simulink library "GOcontroll_Moduline_Target"  (R2023b)
settings: Solver=ode45  StartTime=0.0  StopTime=10.0  RelTol=1e-3  EnableMultiTasking=on
PreLoadFcn:
  | compile_gocontroll_mex;
libraries: $bdroot x8, canmsglib x4, simulink x2
(part 2 of 4)

== system GOcontroll_Moduline_Target/Modules/Bridge Module ==
  Bridge Module : M-S-Function  FunctionName=sfcn_gocontroll_bridge_module  Parameters=tsamp  mask(Bridge Module){tsamp=1, ContrType=GOcontroll Moduline IV, moduleSlot=Moduleslot 1, C1func=Disable (output disabled), C1freq=100 Hz, C2func=Disable (output disabled), C2freq=100 Hz}
      mask prompts: tsamp "Sample time"; ContrType "Controller Type"; moduleSlot "Module Slot"; C1func "Function select"; C1freq "Frequency"; C2func "Function select"; C2freq "Frequency"
      mask help:
      | With this function block, you can configure each output of the bridge module (202001xx). During initialization of the controller, the corresponding outputs of the module are set according the settings. During runtime, the value pushed into the block will control the outputs.
      |
      | Module slot:
      | Sets the location of the module slot where the module is physically
      | plugged into.
      |
      | Channel tabs:
      | Each ouput has its own configuration tab.
      |
      | Function select:
      | Select the desired output configuration.
      |
      | Frequency:
      | In case a duty cycle is used, select the frequency.
      mask init:
      | % array with pinID infos
      | 	moduleSlotInfoStrings = {  	'Module Slot 1',  ...
      | 								'Module Slot 2',  ...
      | 								'Module Slot 3',  ...
      | 								'Module Slot 4',  ...
      | 								'Module Slot 5',  ...
      | 								'Module Slot 6',  ...
      | 								'Module Slot 7',  ...
      | 								'Module Slot 8'};
      | 	% construct the pinID info string
      | 	moduleSlotInfoStr = moduleSlotInfoStrings{moduleSlot};
      | 
      | 
      | 	if(moduleSlot == 1 || moduleSlot == 2)
      | 		connectorId = 'A';
      | 	elseif(moduleSlot == 3 || moduleSlot == 4)
      | 		connectorId = 'B';
      | 	elseif(moduleSlot == 5 || moduleSlot == 6)
      | 		connectorId = 'D';
      | 	else
      | 		connectorId = 'E';
      | 	end
      | 
      | 	if (ContrType == 1) % Moduline IV
      | 		if (mod(moduleSlot,2) == 1) %uneven
      | 			pin1Id = 'Pin 11,12,13';
      | 			pin2Id = 'Pin 17,18,19';
      | 		else
      | 			pin1Id = 'Pin 8,9,10';
      | 			pin2Id = 'Pin 14,15,16';
      | 		end
      | 	elseif(ContrType == 2 || ContrType == 3) % Moduline mini / Moduline display
      | 		if(mod(moduleSlot,2) == 1)
      | 			pin1Id = 'Pin 13,14,15';
      | 			pin2Id = 'Pin 21,22,23';
      | 		else
      | 			pin1Id = 'Pin 10,11,12';
      | 			pin2Id = 'Pin 18,19,20';
      | 		end
      |     end
      |     % register rtw data here because the WriteRTW callback doesn't update
      |     % properly
      |     % Create resource keywords to be reserved in resource database
      | 	modelRTWFields = 	struct('moduleSlot', int2str(moduleSlot),	'C1func', int2str(C1func),'C1freq', int2str(C1freq),...
      | 										'C2func', int2str(C2func),'C2freq', int2str(C2freq));
      | 
      | 	set_param(gcb, 'RTWdata', modelRTWFields);
      mask TypeOptions ContrType: GOcontroll Moduline IV | GOcontroll Moduline Mini | GOcontroll Moduline Display
      mask Callback ContrType:
      | msk = Simulink.Mask.get(gcb);
      | p = msk.getParameter('moduleSlot');
      | 
      | func = get_param(gcb,'ContrType');
      | 
      | if(func == "GOcontroll Moduline IV")
      |     p.TypeOptions = {'Moduleslot 1','Moduleslot 2','Moduleslot 3','Moduleslot 4',...
      |                     'Moduleslot 5','Moduleslot 6','Moduleslot 7','Moduleslot 8'};
      | elseif(func == "GOcontroll Moduline Mini")
      |     p.TypeOptions = {'Moduleslot 1','Moduleslot 2','Moduleslot 3','Moduleslot 4'};
      | elseif (func == "GOcontroll Moduline Display")
      |     p.TypeOptions = {'Moduleslot 1','Moduleslot 2'};
      | end
      mask TypeOptions moduleSlot: Moduleslot 1 | Moduleslot 2 | Moduleslot 3 | Moduleslot 4 | Moduleslot 5 | Moduleslot 6 | Moduleslot 7 | Moduleslot 8
      mask TypeOptions C1func: Disable (output disabled) | Half Bridge duty cycle controlled 0% - 100% duty cycle ( 0 - 1000) | Low side switch  duty cycle controlled 0% - 100% duty cycle (0 - 1000) | High side switch  duty cycle controlled 0% - 100% duty cycle (0 - 1000) | Low side switch On - Off (1-0) | High side switch On - Off (1-0)
      mask TypeOptions C1freq: 100 Hz | 200 Hz | 500 Hz | 1 kHz | 2 kHz | 5 kHz | 10 kHz
      mask TypeOptions C2func: Disable (output disabled) | Half Bridge duty cycle controlled 0% - 100% duty cycle ( 0 - 1000) | Low side switch  duty cycle controlled 0% - 100% duty cycle (0 - 1000) | High side switch  duty cycle controlled 0% - 100% duty cycle (0 - 1000) | Low side switch On - Off (1-0) | High side switch On - Off (1-0)
      mask TypeOptions C2freq: 100 Hz | 200 Hz | 500 Hz | 1 kHz | 2 kHz | 5 kHz | 10 kHz
      mask DialogControl Container4 Prompt: Output 1
      mask DialogControl Container5 Prompt: Output 2
      mask Display:
      | fprintf('Bridge Module\n%s\n\n Controller Connector: %s', moduleSlotInfoStr,connectorId);
      | port_label('input', 1, pin1Id);
      | port_label('input', 2, pin2Id);
      | text(2, 6, ert_linux_target_version());
  Bridge Module Monitor : M-S-Function  FunctionName=sfcn_gocontroll_bridge_module_monitor  Parameters=tsamp  mask(Bridge Module Monitor){tsamp=1, ContrType=GOcontroll Moduline IV, moduleSlot=Moduleslot 1}
      mask prompts: tsamp "Sample time"; ContrType "Controller Type"; moduleSlot "Module Slot"
      mask help:
      | With this function block, you can read parameters from the specified bridge module (202001xx). The block will provide some information about the module such as:
      |
      | Module temperature:
      | The temperature in degrees from the output module.
      |
      | Module ground shift
      | In case the ground connection of the module is poor, the power ground is shifted. The value gives the ground difference in mV and schould be beneath 50 mV
      |
      | Channel current
      | Current related output for each output channel
      mask init:
      | % array with pinID infos
      | 	moduleSlotInfoStrings = {  	'Module slot 1',  ...\
      | 								  'Module slot 2',  ...\
      | 								  'Module slot 3',  ...\
      | 								  'Module slot 4',  ...\
      | 								  'Module slot 5',  ...\
      | 								  'Module slot 6',  ...\
      | 								  'Module slot 7',  ...\
      | 								  'Module slot 8'};
      | 	% construct the pinID info string
      | 	moduleSlotInfoStr = moduleSlotInfoStrings{moduleSlot};
      | 
      | 	if(moduleSlot == 1 || moduleSlot == 2)
      | 		connectorId = 'A';
      | 	elseif(moduleSlot == 3 || moduleSlot == 4)
      | 		connectorId = 'B';
      | 	elseif(moduleSlot == 5 || moduleSlot == 6)
      | 		connectorId = 'D';
      | 	else
      | 		connectorId = 'E';
      | 	end
      | 
      | 	if(ContrType == 1) % Moduline IV
      | 		if(mod(moduleSlot,2) == 1)
      | 			pin1Id = 'Pin 11,12,13';
      | 			pin2Id = 'Pin 17,18,19';
      | 		else
      | 			pin1Id = 'Pin 8,9,10';
      | 			pin2Id = 'Pin 14,15,16';
      | 		end
      | 	elseif(ContrType == 2 || ContrType == 3) % Moduline mini / Moduline display
      | 		if(mod(moduleSlot,2) == 1)
      | 			pin1Id = 'Pin 13,14,15';
      | 			pin2Id = 'Pin 21,22,23';
      | 		else
      | 			pin1Id = 'Pin 10,11,12';
      | 			pin2Id = 'Pin 18,19,20';
      | 		end
      | 	end
      |     % update RTWdata to call WriteRTW again
      | 	modelRTWFields = 	struct('moduleSlot', int2str(moduleSlot));
      | 
      | 	set_param(gcb, 'RTWdata', modelRTWFields);
      mask TypeOptions ContrType: GOcontroll Moduline IV | GOcontroll Moduline Mini | GOcontroll Moduline Display
      mask Callback ContrType:
      | msk = Simulink.Mask.get(gcb);
      |     p = msk.getParameter('moduleSlot');
      |     func = get_param(gcb,'ContrType');
      |     if(func == "GOcontroll Moduline IV")
      |         p.TypeOptions = {'Moduleslot 1','Moduleslot 2','Moduleslot 3','Moduleslot 4',...
      |                         'Moduleslot 5','Moduleslot 6','Moduleslot 7','Moduleslot 8'};
      |     elseif (func == "GOcontroll Moduline Mini")
      |         p.TypeOptions = {'Moduleslot 1','Moduleslot 2','Moduleslot 3','Moduleslot 4'};
      |     elseif (func == "GOcontroll Moduline Display")
      |         p.TypeOptions = {'Moduleslot 1','Moduleslot 2'};
      |     end
      mask TypeOptions moduleSlot: Moduleslot 1 | Moduleslot 2 | Moduleslot 3 | Moduleslot 4 | Moduleslot 5 | Moduleslot 6 | Moduleslot 7 | Moduleslot 8
      mask Display:
      | fprintf('Bridge Module Monitor\n%s\n\n Controller Connector: %s', moduleSlotInfoStr,connectorId);
      | port_label('output', 1, 'Temperature');
      | port_label('output', 2, 'Groundshift');
      | port_label('output', 3, pin1Id);
      | port_label('output', 4, pin2Id);
      | text(2, 6, ert_linux_target_version());

== system GOcontroll_Moduline_Target/Modules/Input Module ==
  Input Module (10 channel) : M-S-Function  FunctionName=sfcn_gocontroll_input_module_10  Parameters=tsamp  mask(Input Module){tsamp=0.1, ContrType=GOcontroll Moduline IV, moduleSlot=Moduleslot 1, SensSup1=Supply output enabled, SensSup2=Supply output enabled, C1func=Analog input -  decimal (12 bit resolution), C1pu=no pull up, C1pd=no pull down, C2func=Analog input -  decimal (12 bit resolution), C2pu=no pull up, C2pd=no pull down, C3func=Analog input -  decimal (12 bit resolution), C3pu=no pull up, C3pd=no pull down, C4func=Analog input -  decimal (12 bit resolution), C4pu=no pull up, C4pd=no pull down, C5func=Analog input -  decimal (12 bit resolution), C5pu=no pull up, C5pd=no pull down, C6func=Analog input -  decimal (12 bit resolution), C6pu=no pull up, C6pd=no pull down, C7func=Analog input -  decimal (12 bit resolution), C7pu=no pull up, C7pd=no pull down, C8func=Analog input -  decimal (12 bit resolution), C8pu=no pull up, C8pd=no pull down, C9func=Analog input -  decimal (12 bit resolution), C9pu=no pull up, C9pd=no pull down, C10func=Analog input -  decimal (12 bit resolution), C10pu=no pull up, C10pd=no pull down}
      mask prompts: tsamp "Sample time"; ContrType "Controller Type"; moduleSlot "Module Slot"; SensSup1 "5V Sensor Supply 1"; SensSup2 "5V Sensor Supply 2"; C1func "Function select"; C1pu "Pull up on input"; C1pd "Pull down on input"; C2func "Function select"; C2pu "Pull up on input"; C2pd "Pull down on input"; C3func "Function select"; C3pu "Pull up on input"; C3pd "Pull down on input"; C4func "Function select"; C4pu "Pull up on input"; C4pd "Pull down on input"; C5func "Function select"; C5pu "Pull up on input"; C5pd "Pull down on input"; C6func "Function select"; C6pu "Pull up on input"; C6pd "Pull down on input"; C7func "Function select"; C7pu "Pull up on input"; C7pd "Pull down on input"; C8func "Function select"; C8pu "Pull up on input"; C8pd "Pull down on input"; C9func "Function select"; C9pu "Pull up on input"; C9pd "Pull down on input"; C10func "Function select"; C10pu "Pull up on input"; C10pd "Pull down on input"
      mask help:
      | With this block, you can configure each channel of the 10 channel input module (201002xx). The configuration of the module is set once at initialization. During runtime, the block outputs the measured values from each channel.
      |
      | Module location:
      | Sets the location of the module slot where the module is physically
      | plugged into.
      |
      | Channel tabs:
      | Each channel has its own configuration tab.
      |
      | Function select:
      | Select the desired input signal configuration.
      |
      | Pull Up:
      | If required, a pull-up resistance can be added to the input signal.
      |
      | Pull Down:
      | If required, a pull-down resistance can be added to the input signal.
      mask init:
      | % array with module slot infos
      | moduleSlotInfoStrings = {  	'Module slot 1',  ...\
      | 							'Module slot 2',  ...\
      | 							'Module slot 3',  ...\
      | 							'Module slot 4',  ...\
      | 							'Module slot 5',  ...\
      | 							'Module slot 6',  ...\
      | 							'Module slot 7',  ...\
      | 							'Module slot 8'};
      | 
      | % construct the module slot info string
      | moduleSlotInfoStr = moduleSlotInfoStrings{moduleSlot};
      | 
      | if(moduleSlot == 1 || moduleSlot == 2)
      | connectorId = 'A';
      | elseif(moduleSlot == 3 || moduleSlot == 4)
      | connectorId = 'B';
      | elseif(moduleSlot == 5 || moduleSlot == 6)
      | connectorId = 'D';
      | else
      | connectorId = 'E';
      | end
      | 
      | if(ContrType == 1) % Moduline IV
      | 	if(moduleSlot == 1 || moduleSlot == 3 || moduleSlot == 5 || moduleSlot == 7)
      | 		pin1Id = 'Pin 13';
      | 		pin2Id = 'Pin 19';
      | 		pin3Id = 'Pin 12';
      | 		pin4Id = 'Pin 18';
      | 		pin5Id = 'Pin 11';
      | 		pin6Id = 'Pin 17';
      | 		pin7Id = 'Pin 25';
      | 		pin8Id = 'Pin 24';
      | 		pin9Id = 'Pin 5';
      | 		pin10Id = 'Pin 4';
      | 	else
      | 		pin1Id = 'Pin 8';
      | 		pin2Id = 'Pin 14';
      | 		pin3Id = 'Pin 9';
      | 		pin4Id = 'Pin 15';
      | 		pin5Id = 'Pin 10';
      | 		pin6Id = 'Pin 16';
      | 		pin7Id = 'Pin 21';
      | 		pin8Id = 'Pin 22';
      | 		pin9Id = 'Pin 3';
      | 		pin10Id = 'Pin 23';
      | 	end
      | elseif(ContrType == 2 || ContrType == 3) % Moduline mini / Moduline display
      | 	if(moduleSlot == 1 || moduleSlot == 3)
      | 		pin1Id = 'Pin 15';
      | 		pin2Id = 'Pin 23';
      | 		pin3Id = 'Pin 14';
      | 		pin4Id = 'Pin 22';
      | 		pin5Id = 'Pin 13';
      | 		pin6Id = 'Pin 21';
      | 		pin7Id = 'Pin 31';
      | 		pin8Id = 'Pin 30';
      | 		pin9Id = 'Pin 5';
      | 		pin10Id = 'Pin 4';
      | 	else
      | 		pin1Id = 'Pin 10';
      | 		pin2Id = 'Pin 18';
      | 		pin3Id = 'Pin 11';
      | 		pin4Id = 'Pin 19';
      | 		pin5Id = 'Pin 12';
      | 		pin6Id = 'Pin 20';
      | 		pin7Id = 'Pin 27';
      | 		pin8Id = 'Pin 28';
      | 		pin9Id = 'Pin 3';
      | 		pin10Id = 'Pin 29';
      | 	end
      | end
      | 
      | % Create resource keywords to be reserved in resource database
      | modelRTWFields = struct('moduleSlot', int2str(moduleSlot),	'C1func',int2str(C1func),'C1pu', int2str(C1pu),'C1pd', int2str(C1pd),...
      | 															'C2func', int2str(C2func),'C2pu', int2str(C2pu),'C2pd', int2str(C2pd),...
      | 															'C3func', int2str(C3func),'C3pu', int2str(C3pu),'C3pd', int2str(C3pd),...
      | 															'C4func', int2str(C4func),'C4pu', int2str(C4pu),'C4pd', int2str(C4pd),...
      | 															'C5func', int2str(C5func),'C5pu', int2str(C5pu),'C5pd', int2str(C5pd),...
      | 															'C6func', int2str(C6func),'C6pu', int2str(C6pu),'C6pd', int2str(C6pd),...
      | 															'C7func', int2str(C7func),'C7pu', int2str(C7pu),'C7pd', int2str(C7pd),...
      | 															'C8func', int2str(C8func),'C8pu', int2str(C8pu),'C8pd', int2str(C8pd),...
      | 															'C9func', int2str(C9func),'C9pu', int2str(C9pu),'C9pd', int2str(C9pd),...
      | 															'C10func', int2str(C10func),'C10pu', int2str(C10pu),'C10pd', int2str(C10pd),...
      | 															'SensSup1', int2str(SensSup1), 'SensSup2', int2str(SensSup2));
      | 
      | set_param(gcb, 'RTWdata', modelRTWFields);
      mask TypeOptions ContrType: GOcontroll Moduline IV | GOcontroll Moduline Mini | GOcontroll Moduline Display
      mask Callback ContrType:
      | msk = Simulink.Mask.get(gcb);
      | slot_param = msk.getParameter('moduleSlot');
      | 
      | func = get_param(gcb,'ContrType');
      | 
      | if(func == "GOcontroll Moduline IV")
      |     slot_param.TypeOptions = {'Moduleslot 1','Moduleslot 2','Moduleslot 3','Moduleslot 4',...
      |                     'Moduleslot 5','Moduleslot 6','Moduleslot 7','Moduleslot 8'};
      | elseif (func == "GOcontroll Moduline Mini")
      |     slot_param.TypeOptions = {'Moduleslot 1','Moduleslot 2','Moduleslot 3','Moduleslot 4'};
      | elseif (func == "GOcontroll Moduline Display")
      |     slot_param.TypeOptions = {'Moduleslot 1','Moduleslot 2'};
      | end
      mask TypeOptions moduleSlot: Moduleslot 1 | Moduleslot 2 | Moduleslot 3 | Moduleslot 4 | Moduleslot 5 | Moduleslot 6 | Moduleslot 7 | Moduleslot 8
      mask TypeOptions SensSup1: Supply output enabled | Supply output disabled
      mask TypeOptions SensSup2: Supply output enabled | Supply output disabled
      mask TypeOptions C1func: Analog input -  decimal (12 bit resolution) | Analog input -  mV (1mV resolution) | Digital input - status (high or low) | Digital input - frequency (1Hz to 10 kHz) | Digital input - duty cycle low time (0.1% resolution) | Digital input - duty cycle high time (0.1% resolution) | Digital input - rotation speed (rpm) | Digital input - pulse counter (in combination with channel 2)
      mask TypeOptions C1pu: no pull up | 10 K ohm
      mask TypeOptions C1pd: no pull down | 3,3 K ohm
      mask TypeOptions C2func: Analog input -  decimal (12 bit resolution) | Analog input -  mV (1mV resolution) | Digital input - status (high or low) | Digital input - frequency (1Hz to 10 kHz) | Digital input - duty cycle low time (0.1% resolution) | Digital input - duty cycle high time (0.1% resolution) | Digital input - rotation speed (rpm) | Digital input - pulse counter (in combination with channel 1)
      mask TypeOptions C2pu: no pull up | 10 K ohm
      mask TypeOptions C2pd: no pull down | 3,3 K ohm
      mask TypeOptions C3func: Analog input -  decimal (12 bit resolution) | Analog input -  mV (1mV resolution) | Digital input - status (high or low) | Digital input - frequency (1Hz to 10 kHz) | Digital input - duty cycle low time (0.1% resolution) | Digital input - duty cycle high time (0.1% resolution) | Digital input - rotation speed (rpm) | Digital input - pulse counter (in combination with channel 4)
      mask TypeOptions C3pu: no pull up | 10 K ohm
      mask TypeOptions C3pd: no pull down | 3,3 K ohm
      mask TypeOptions C4func: Analog input -  decimal (12 bit resolution) | Analog input -  mV (1mV resolution) | Digital input - status (high or low) | Digital input - frequency (1Hz to 10 kHz) | Digital input - duty cycle low time (0.1% resolution) | Digital input - duty cycle high time (0.1% resolution) | Digital input - rotation speed (rpm) | Digital input - pulse counter (in combination with channel 3)
      mask TypeOptions C4pu: no pull up | 10 K ohm
      mask TypeOptions C4pd: no pull down | 3,3 K ohm
      mask TypeOptions C5func: Analog input -  decimal (12 bit resolution) | Analog input -  mV (1mV resolution) | Digital input - status (high or low) | Digital input - frequency (1Hz to 10 kHz) | Digital input - duty cycle low time (0.1% resolution) | Digital input - duty cycle high time (0.1% resolution) | Digital input - rotation speed (rpm) | Digital input - pulse counter (in combination with channel 6)
      mask TypeOptions C5pu: no pull up | 10 K ohm
      mask TypeOptions C5pd: no pull down | 3,3 K ohm
      mask TypeOptions C6func: Analog input -  decimal (12 bit resolution) | Analog input -  mV (1mV resolution) | Digital input - status (high or low) | Digital input - frequency (1Hz to 10 kHz) | Digital input - duty cycle low time (0.1% resolution) | Digital input - duty cycle high time (0.1% resolution) | Digital input - rotation speed (rpm) | Digital input - pulse counter (in combination with channel 5)
      mask TypeOptions C6pu: no pull up | 10 K ohm
      mask TypeOptions C6pd: no pull down | 3,3 K ohm
      mask TypeOptions C7func: Analog input -  decimal (12 bit resolution) | Analog input -  mV (1mV resolution) | Digital input - status (high or low) | Digital input - frequency (1Hz to 10 kHz) | Digital input - duty cycle low time (0.1% resolution) | Digital input - duty cycle high time (0.1% resolution) | Digital input - rotation speed (rpm) | Digital input - pulse counter (in combination with channel 8)
      mask TypeOptions C7pu: no pull up | 10 K ohm
      mask TypeOptions C7pd: no pull down | 3,3 K ohm
      mask TypeOptions C8func: Analog input -  decimal (12 bit resolution) | Analog input -  mV (1mV resolution) | Digital input - status (high or low) | Digital input - frequency (1Hz to 10 kHz) | Digital input - duty cycle low time (0.1% resolution) | Digital input - duty cycle high time (0.1% resolution) | Digital input - rotation speed (rpm) | Digital input - pulse counter (in combination with channel 7)
      mask TypeOptions C8pu: no pull up | 10 K ohm
      mask TypeOptions C8pd: no pull down | 3,3 K ohm
      mask TypeOptions C9func: Analog input -  decimal (12 bit resolution) | Analog input -  mV (1mV resolution) | Digital input - status (high or low) | Digital input - frequency (1Hz to 10 kHz) | Digital input - duty cycle low time (0.1% resolution) | Digital input - duty cycle high time (0.1% resolution) | Digital input - rotation speed (rpm) | Digital input - pulse counter (in combination with channel 10)
      mask TypeOptions C9pu: no pull up | 10 K ohm
      mask TypeOptions C9pd: no pull down | 3,3 K ohm
      mask TypeOptions C10func: Analog input -  decimal (12 bit resolution) | Analog input -  mV (1mV resolution) | Digital input - status (high or low) | Digital input - frequency (1Hz to 10 kHz) | Digital input - duty cycle low time (0.1% resolution) | Digital input - duty cycle high time (0.1% resolution) | Digital input - rotation speed (rpm) | Digital input - pulse counter (in combination with channel 9)
      mask TypeOptions C10pu: no pull up | 10 K ohm
      mask TypeOptions C10pd: no pull down | 3,3 K ohm
      mask DialogControl Container4 Prompt: Input 1
      mask DialogControl Container5 Prompt: Input 2
      mask DialogControl Container8 Prompt: Input 3
      mask DialogControl Container9 Prompt: Input 4
      mask DialogControl Container7 Prompt: Input 5
      mask DialogControl Container12 Prompt: Input 6
      mask DialogControl Container6 Prompt: Input 7
      mask DialogControl Container10 Prompt: Input 8
      mask DialogControl Container11 Prompt: Input 9
      mask DialogControl Container13 Prompt: Input 10
      mask Display:
      | fprintf('10 Channel Input Module \n%s\n\n Controller Connector: %s', moduleSlotInfoStr,connectorId);
      | port_label('output', 1, pin1Id);
      | port_label('output', 2, pin2Id);
      | port_label('output', 3, pin3Id);
      | port_label('output', 4, pin4Id);
      | port_label('output', 5, pin5Id);
      | port_label('output', 6, pin6Id);
      | port_label('output', 7, pin7Id);
      | port_label('output', 8, pin8Id);
      | port_label('output', 9, pin9Id);
      | port_label('output', 10, pin10Id);
      | text(2, 6, ert_linux_target_version());
  Input Module (6 channel) : M-S-Function  FunctionName=sfcn_gocontroll_input_module  Parameters=tsamp  mask(Input Module){tsamp=0.1, ContrType=GOcontroll Moduline IV, moduleSlot=Moduleslot 1, SensSup1=Supply output enabled, SensSup2=Supply output enabled, SensSup3=Supply output enabled, C1func=Analog input -  decimal (12 bit resolution), C1volt=0 - 5 V, C1afil=0, C1dpul=1, C1pu=no pull up, C1pd=no pull down, C2func=Analog input -  decimal (12 bit resolution), C2volt=0 - 5 V, C2afil=0, C2dpul=1, C2pu=no pull up, C2pd=no pull down, C3func=Analog input -  decimal (12 bit resolution), C3volt=0 - 5 V, C3afil=0, C3dpul=1, C3pu=no pull up, C3pd=no pull down, C4func=Analog input -  decimal (12 bit resolution), C4volt=0 - 5 V, C4afil=0, C4dpul=1, C4pu=no pull up, C4pd=no pull down, C5func=Analog input -  decimal (12 bit resolution), C5volt=0 - 5 V, C5afil=0, C5dpul=1, C5pu=no pull up, C5pd=no pull down, C6func=Analog input -  decimal (12 bit resolution), C6volt=0 - 5 V, C6afil=0, C6dpul=1, C6pu=no pull up, C6pd=no pull down}
      mask prompts: tsamp "Sample time"; ContrType "Controller Type"; moduleSlot "Module Slot"; SensSup1 "5V Sensor Supply 1"; SensSup2 "5V Sensor Supply 2"; SensSup3 "5V Sensor Supply 3"; C1func "Function select"; C1volt "Voltage range"; C1afil "Analog filter samples (0 - 1000)"; C1dpul "Pulses per rotation (1-200)"; C1pu "Pull up on input"; C1pd "Pull down on input"; C2func "Function select"; C2volt "Voltage range"; C2afil "Analog filter samples (0 - 1000)"; C2dpul "Pulses per rotation (1-200)"; C2pu "Pull up on input"; C2pd "Pull down on input"; C3func "Function select"; C3volt "Voltage range"; C3afil "Analog filter samples (0 - 1000)"; C3dpul "Pulses per rotation (1-200)"; C3pu "Pull up on input"; C3pd "Pull down on input"; C4func "Function select"; C4volt "Voltage range"; C4afil "Analog filter samples (0 - 1000)"; C4dpul "Pulses per rotation (1-200)"; C4pu "Pull up on input"; C4pd "Pull down on input"; C5func "Function select"; C5volt "Voltage range"; C5afil "Analog filter samples (0 - 1000)"; C5dpul "Pulses per rotation (1-200)"; C5pu "Pull up on input"; C5pd "Pull down on input"; C6func "Function select"; C6volt "Voltage range"; C6afil "Analog filter samples (0 - 1000)"; C6dpul "Pulses per rotation (1-200)"; C6pu "Pull up on input"; C6pd "Pull down on input"
      mask help:
      | With this function block, you can configure each channel of the 6 channel input module (201001xx). The configuration of the module is set once at initialization. During runtime, the block outputs the measured values from each channel.
      |
      | Module location:
      | Sets the location of the module slot where the module is physically
      | plugged into.
      |
      | Channel tabs:
      | Each channel has its own configuration tab.
      |
      | Function select:
      | Select the desired input signal configuration.
      |
      | Voltage range:
      | Select the expected input range of the signal.
      |
      | Analog filter samples:
      | The number of samples that are passed into a moving average filter.
      | (only active in case of an analog input)
      |
      | Pulses per rotation
      | The number of pulses for one rotation. This parameter is needed in case the
      | module needs to calculate the rotation speed from i.e. an axle.
      |
      | Pull Up:
      | If required, a pull-up resistance can be added to the input signal.
      |
      | Pull Down:
      | If required, a pull-down resistance can be added to the input signal.
      mask init:
      | % array with module slot infos
      |   moduleSlotInfoStrings = {  	'Module slot 1',  ...\
      | 								'Module slot 2',  ...\
      | 								'Module slot 3',  ...\
      | 								'Module slot 4',  ...\
      | 								'Module slot 5',  ...\
      | 								'Module slot 6',  ...\
      | 								'Module slot 7',  ...\
      | 								'Module slot 8'};
      | 
      |   % construct the module slot info string
      |   moduleSlotInfoStr = moduleSlotInfoStrings{moduleSlot};
      | 
      |     if(moduleSlot == 1 || moduleSlot == 2)
      | 	    connectorId = 'A';
      |     elseif(moduleSlot == 3 || moduleSlot == 4)
      | 	    connectorId = 'B';
      |     elseif(moduleSlot == 5 || moduleSlot == 6)
      | 	    connectorId = 'D';
      |     else
      | 	    connectorId = 'E';
      |     end
      |     
      |     
      |     if(ContrType == 1) % Moduline IV
      | 	    if(moduleSlot == 1 || moduleSlot == 3 || moduleSlot == 5 || moduleSlot == 7)
      | 		    pin1Id = 'Pin 13';
      | 		    pin2Id = 'Pin 19';
      | 		    pin3Id = 'Pin 12';
      | 		    pin4Id = 'Pin 18';
      | 		    pin5Id = 'Pin 11';
      | 		    pin6Id = 'Pin 17';
      | 	    else
      | 		    pin1Id = 'Pin 8';
      | 		    pin2Id = 'Pin 14';
      | 		    pin3Id = 'Pin 9';
      | 		    pin4Id = 'Pin 15';
      | 		    pin5Id = 'Pin 10';
      | 		    pin6Id = 'Pin 16';
      | 	    end
      |     elseif(ContrType == 2 || ContrType == 3) % Moduline mini / Moduline display
      | 	    if(moduleSlot == 1 || moduleSlot == 3)
      | 		    pin1Id = 'Pin 15';
      | 		    pin2Id = 'Pin 23';
      | 		    pin3Id = 'Pin 14';
      | 		    pin4Id = 'Pin 22';
      | 		    pin5Id = 'Pin 13';
      | 		    pin6Id = 'Pin 21';
      | 	    else
      | 		    pin1Id = 'Pin 10';
      | 		    pin2Id = 'Pin 18';
      | 		    pin3Id = 'Pin 11';
      | 		    pin4Id = 'Pin 19';
      | 		    pin5Id = 'Pin 12';
      | 		    pin6Id = 'Pin 20';
      | 	    end
      |     end
      |     
      |     % Update RTWdata
      |     modelRTWFields = struct('moduleSlot', int2str(moduleSlot),	'C1func', int2str(C1func),'C1volt', int2str(C1volt), 'C1afil', int2str(C1afil),'C1dpul', int2str(C1dpul),'C1pu', int2str(C1pu),'C1pd', int2str(C1pd),...
      | 															    'C2func', int2str(C2func),'C2volt', int2str(C2volt), 'C2afil', int2str(C2afil),'C2dpul', int2str(C2dpul),'C2pu', int2str(C2pu),'C2pd', int2str(C2pd),...
      | 															    'C3func', int2str(C3func),'C3volt', int2str(C3volt), 'C3afil', int2str(C3afil),'C3dpul', int2str(C3dpul),'C3pu', int2str(C3pu),'C3pd', int2str(C3pd),...
      | 															    'C4func', int2str(C4func),'C4volt', int2str(C4volt), 'C4afil', int2str(C4afil),'C4dpul', int2str(C4dpul),'C4pu', int2str(C4pu),'C4pd', int2str(C4pd),...
      | 															    'C5func', int2str(C5func),'C5volt', int2str(C5volt), 'C5afil', int2str(C5afil),'C5dpul', int2str(C5dpul),'C5pu', int2str(C5pu),'C5pd', int2str(C5pd),...
      | 															    'C6func', int2str(C6func),'C6volt', int2str(C6volt), 'C6afil', int2str(C6afil),'C6dpul', int2str(C6dpul),'C6pu', int2str(C6pu),'C6pd', int2str(C6pd),...
      | 															    'SensSup1', int2str(SensSup1),'SensSup2', int2str(SensSup2), 'SensSup3', int2str(SensSup3));
      | 
      |     set_param(gcb, 'RTWdata', modelRTWFields);
      mask TypeOptions ContrType: GOcontroll Moduline IV | GOcontroll Moduline Mini | GOcontroll Moduline Display
      mask Callback ContrType:
      | msk = Simulink.Mask.get(gcb);
      | p = msk.getParameter('moduleSlot');
      | 
      | func = get_param(gcb,'ContrType');
      | 
      | if(func == "GOcontroll Moduline IV")
      |     p.TypeOptions = {'Moduleslot 1','Moduleslot 2','Moduleslot 3','Moduleslot 4',...
      |                     'Moduleslot 5','Moduleslot 6','Moduleslot 7','Moduleslot 8'};
      | elseif (func == "GOcontroll Moduline Mini")
      |     p.TypeOptions = {'Moduleslot 1','Moduleslot 2','Moduleslot 3','Moduleslot 4'};
      | elseif (func == "GOcontroll Moduline Display")
      |     p.TypeOptions = {'Moduleslot 1','Moduleslot 2'};
      | end
      mask TypeOptions moduleSlot: Moduleslot 1 | Moduleslot 2 | Moduleslot 3 | Moduleslot 4 | Moduleslot 5 | Moduleslot 6 | Moduleslot 7 | Moduleslot 8
      mask TypeOptions SensSup1: Supply output enabled | Supply output disabled
      mask TypeOptions SensSup2: Supply output enabled | Supply output disabled
      mask TypeOptions SensSup3: Supply output enabled | Supply output disabled
      mask TypeOptions C1func: Analog input -  decimal (12 bit resolution) | Analog input -  mV (1mV resolution) | Digital input - status (high or low) | Digital input - frequency (1Hz to 10 kHz) | Digital input - duty cycle low time (0.1% resolution) | Digital input - duty cycle high time (0.1% resolution) | Digital input - rotation speed (rpm) | Digital input - pulse counter (in combination with channel 2)
      mask TypeOptions C1volt: 0 - 5 V | 0 - 10V (external sensor supply) | 0 - 24V (external sensor supply)
      mask TypeOptions C1pu: no pull up | 3,3 K ohm | 4,7 K ohm | 10 K ohm
      mask TypeOptions C1pd: no pull down | 3,3 K ohm | 4,7 K ohm | 10 K ohm
      mask TypeOptions C2func: Analog input -  decimal (12 bit resolution) | Analog input -  mV (1mV resolution) | Digital input - status (high or low) | Digital input - frequency (1Hz to 10 kHz) | Digital input - duty cycle low time (0.1% resolution) | Digital input - duty cycle high time (0.1% resolution) | Digital input - rotation speed (rpm) | Digital input - pulse counter (in combination with channel 1)
      mask TypeOptions C2volt: 0 - 5 V | 0 - 10V (external sensor supply) | 0 - 24V (external sensor supply)
      mask TypeOptions C2pu: no pull up | 3,3 K ohm | 4,7 K ohm | 10 K ohm
      mask TypeOptions C2pd: no pull down | 3,3 K ohm | 4,7 K ohm | 10 K ohm
      mask TypeOptions C3func: Analog input -  decimal (12 bit resolution) | Analog input -  mV (1mV resolution) | Digital input - status (high or low) | Digital input - frequency (1Hz to 10 kHz) | Digital input - duty cycle low time (0.1% resolution) | Digital input - duty cycle high time (0.1% resolution) | Digital input - rotation speed (rpm) | Digital input - pulse counter (in combination with channel 4)
      mask TypeOptions C3volt: 0 - 5 V | 0 - 10V (external sensor supply) | 0 - 24V (external sensor supply)
      mask TypeOptions C3pu: no pull up | 3,3 K ohm | 4,7 K ohm | 10 K ohm
      mask TypeOptions C3pd: no pull down | 3,3 K ohm | 4,7 K ohm | 10 K ohm
      mask TypeOptions C4func: Analog input -  decimal (12 bit resolution) | Analog input -  mV (1mV resolution) | Digital input - status (high or low) | Digital input - frequency (1Hz to 10 kHz) | Digital input - duty cycle low time (0.1% resolution) | Digital input - duty cycle high time (0.1% resolution) | Digital input - rotation speed (rpm) | Digital input - pulse counter (in combination with channel 3) | TFmini plus - Benewake LIDAR sensor
      mask TypeOptions C4volt: 0 - 5 V | 0 - 10V (external sensor supply) | 0 - 24V (external sensor supply)
      mask TypeOptions C4pu: no pull up | 3,3 K ohm | 4,7 K ohm | 10 K ohm
      mask TypeOptions C4pd: no pull down | 3,3 K ohm | 4,7 K ohm | 10 K ohm
      mask TypeOptions C5func: Analog input -  decimal (12 bit resolution) | Analog input -  mV (1mV resolution) | Digital input - status (high or low) | Digital input - frequency (1Hz to 10 kHz) | Digital input - duty cycle low time (0.1% resolution) | Digital input - duty cycle high time (0.1% resolution) | Digital input - rotation speed (rpm) | Digital input - pulse counter (in combination with channel 6)
      mask TypeOptions C5volt: 0 - 5 V | 0 - 10V (external sensor supply) | 0 - 24V (external sensor supply)
      mask TypeOptions C5pu: no pull up | 3,3 K ohm | 4,7 K ohm | 10 K ohm
      mask TypeOptions C5pd: no pull down | 3,3 K ohm | 4,7 K ohm | 10 K ohm
      mask TypeOptions C6func: Analog input -  decimal (12 bit resolution) | Analog input -  mV (1mV resolution) | Digital input - status (high or low) | Digital input - frequency (1Hz to 10 kHz) | Digital input - duty cycle low time (0.1% resolution) | Digital input - duty cycle high time (0.1% resolution) | Digital input - rotation speed (rpm) | Digital input - pulse counter (in combination with channel 5)
      mask TypeOptions C6volt: 0 - 5 V | 0 - 10V (external sensor supply) | 0 - 24V (external sensor supply)
      mask TypeOptions C6pu: no pull up | 3,3 K ohm | 4,7 K ohm | 10 K ohm
      mask TypeOptions C6pd: no pull down | 3,3 K ohm | 4,7 K ohm | 10 K ohm
      mask DialogControl Container4 Prompt: Input 1
      mask DialogControl Container5 Prompt: Input 2
      mask DialogControl Container8 Prompt: Input 3
      mask DialogControl Container9 Prompt: Input 4
      mask DialogControl Container7 Prompt: Input 5
      mask DialogControl Container12 Prompt: Input 6
      mask Display:
      | fprintf('6 Channel Input Module \n%s\n\n Controller Connector: %s', moduleSlotInfoStr,connectorId);
      | port_label('output', 1, pin1Id);
      | port_label('output', 2, pin2Id);
      | port_label('output', 3, pin3Id);
      | port_label('output', 4, pin4Id);
      | port_label('output', 5, pin5Id);
      | port_label('output', 6, pin6Id);
      | text(2, 6, ert_linux_target_version());
  Input Module 4-20 mA (10 channel) : M-S-Function  FunctionName=sfcn_gocontroll_input_module_420ma  Parameters=tsamp  mask(4-20 mA Input Module){tsamp=0.1, ContrType=GOcontroll Moduline IV, moduleSlot=Moduleslot 1, Sup16ch12=Supply enabled, Sup16ch34=Supply enabled, Sup16ch56=Supply enabled, Sup16ch78=Supply enabled, Sup16ch910=Supply enabled}
      mask prompts: tsamp "Sample time"; ContrType "Controller type"; moduleSlot "Module slot"; Sup16ch12 "Supply channel 1 and 2"; Sup16ch34 "Supply channel 3 and 4"; Sup16ch56 "Supply channel 5 and 6"; Sup16ch78 "Supply channel 7 and 8"; Sup16ch910 "Supply channel 9 and 10"
      mask help:
      | Controller type:
      | Selects the controller that is to be programmed. Pinning on the mask will be adopted accordingly.
      |
      | Module slot:
      | Sets the location of the module slot where the module is physically plugged into.
      |
      | Supply for different channels:
      | Enables the 16V supply per 2 channels. When some input pins are not used, it is recommended to disable these inputs to prevent controller pins floating at 16V.
      |
      | Module status:
      | The status output provides information of the actual state per 2 channels:
      |
      | 0x00 all channels are supplied no problems.
      | 0x01 Channel 1 & 2 over current detected and supply disconnected.
      | 0x02 Channel 3 & 4 over current detected and supply disconnected.
      | 0x04 Channel 5 & 6 over current detected and supply disconnected.
      | 0x08 Channel 7 & 8 over current detected and supply disconnected.
      | 0x10 Channel 9 & 10 over current detected and supply disconnected.
      mask init:
      | % array with module slot infos
      | moduleSlotInfoStrings = {	'Module slot 1',  ...\
      | 							'Module slot 2',  ...\
      | 							'Module slot 3',  ...\
      | 							'Module slot 4',  ...\
      | 							'Module slot 5',  ...\
      | 							'Module slot 6',  ...\
      | 							'Module slot 7',  ...\
      | 							'Module slot 8'};
      | 
      | % construct the module slot info string
      | moduleSlotInfoStr = moduleSlotInfoStrings{moduleSlot};
      | 
      | if(moduleSlot == 1 || moduleSlot == 2)
      | connectorId = 'A';
      | elseif(moduleSlot == 3 || moduleSlot == 4)
      | connectorId = 'B';
      | elseif(moduleSlot == 5 || moduleSlot == 6)
      | connectorId = 'D';
      | else
      | connectorId = 'E';
      | end
      | 
      | if(ContrType == 1) % Moduline IV
      | 	if(moduleSlot == 1 || moduleSlot == 3 || moduleSlot == 5 || moduleSlot == 7)
      | 		pin1Id = 'Pin 7';
      | 		pin2Id = 'Pin 13';
      | 		pin3Id = 'Pin 19';
      | 		pin4Id = 'Pin 6';
      | 		pin5Id = 'Pin 12';
      | 		pin6Id = 'Pin 18';
      | 		pin7Id = 'Pin 5';
      | 		pin8Id = 'Pin 11';
      | 		pin9Id = 'Pin 17';
      | 		pin10Id = 'Pin 4';
      | 	else
      | 		pin1Id = 'Pin 1';
      | 		pin2Id = 'Pin 8';
      | 		pin3Id = 'Pin 14';
      | 		pin4Id = 'Pin 2';
      | 		pin5Id = 'Pin 9';
      | 		pin6Id = 'Pin 15';
      | 		pin7Id = 'Pin 3';
      | 		pin8Id = 'Pin 10';
      | 		pin9Id = 'Pin 16';
      | 		pin10Id = 'Pin 23';
      | 	end
      | elseif(ContrType == 2 || ContrType == 3) % Moduline mini / Moduline display
      | 	if(moduleSlot == 1 || moduleSlot == 3)
      | 		pin1Id = 'Pin 7';
      | 		pin2Id = 'Pin 15';
      | 		pin3Id = 'Pin 23';
      | 		pin4Id = 'Pin 6';
      | 		pin5Id = 'Pin 14';
      | 		pin6Id = 'Pin 22';
      | 		pin7Id = 'Pin 5';
      | 		pin8Id = 'Pin 13';
      | 		pin9Id = 'Pin 21';
      | 		pin10Id = 'Pin 4';
      | 	else
      | 		pin1Id = 'Pin 1';
      | 		pin2Id = 'Pin 10';
      | 		pin3Id = 'Pin 18';
      | 		pin4Id = 'Pin 2';
      | 		pin5Id = 'Pin 11';
      | 		pin6Id = 'Pin 19';
      | 		pin7Id = 'Pin 3';
      | 		pin8Id = 'Pin 12';
      | 		pin9Id = 'Pin 20';
      | 		pin10Id = 'Pin 29';
      | 	end
      | end
      | 
      | % Create resource keywords to be reserved in resource database
      | modelRTWFields = struct('moduleSlot', int2str(moduleSlot),...
      | 						'Sup16ch12', int2str(Sup16ch12),'Sup16ch34', int2str(Sup16ch34),'Sup16ch56', int2str(Sup16ch56),...
      |                         'Sup16ch78', int2str(Sup16ch78),'Sup16ch910', int2str(Sup16ch910));
      | 
      | set_param(gcb, 'RTWdata', modelRTWFields);
      mask TypeOptions ContrType: GOcontroll Moduline IV | GOcontroll Moduline Mini | GOcontroll Moduline Display
      mask Callback ContrType:
      | msk = Simulink.Mask.get(gcb);
      | p = msk.getParameter('moduleSlot');
      | 
      | func = get_param(gcb,'ContrType');
      | 
      | if(func == "GOcontroll Moduline IV")
      | p.TypeOptions = {'Moduleslot 1','Moduleslot 2','Moduleslot 3','Moduleslot 4',...
      |                     'Moduleslot 5','Moduleslot 6','Moduleslot 7','Moduleslot 8'};
      | elseif (func == "GOcontroll Moduline Mini")
      |     p.TypeOptions = {'Moduleslot 1','Moduleslot 2','Moduleslot 3','Moduleslot 4'};
      | elseif (func == "GOcontroll Moduline Display")
      |     p.TypeOptions = {'Moduleslot 1','Moduleslot 2'};
      | end
      mask TypeOptions moduleSlot: Moduleslot 1 | Moduleslot 2 | Moduleslot 3 | Moduleslot 4 | Moduleslot 5 | Moduleslot 6 | Moduleslot 7 | Moduleslot 8
      mask TypeOptions Sup16ch12: Supply disabled | Supply enabled
      mask TypeOptions Sup16ch34: Supply disabled | Supply enabled
      mask TypeOptions Sup16ch56: Supply disabled | Supply enabled
      mask TypeOptions Sup16ch78: Supply disabled | Supply enabled
      mask TypeOptions Sup16ch910: Supply disabled | Supply enabled
      mask Display:
      | fprintf('4-20 mA Input Module \n%s\n\n Controller Connector: %s', moduleSlotInfoStr,connectorId);
      | port_label('output', 1, "Status");
      | port_label('output', 2, pin1Id);
      | port_label('output', 3, pin2Id);
      | port_label('output', 4, pin3Id);
      | port_label('output', 5, pin4Id);
      | port_label('output', 6, pin5Id);
      | port_label('output', 7, pin6Id);
      | port_label('output', 8, pin7Id);
      | port_label('output', 9, pin8Id);
      | port_label('output', 10, pin9Id);
      | port_label('output', 11, pin10Id);
      | text(2, 6, ert_linux_target_version());
  Reset Pulse Counter (6 channel) : M-S-Function  FunctionName=sfcn_gocontroll_input_module_reset  Parameters=tsamp  mask(Reset pulse counter){tsamp=-1, contrType=GOcontroll Moduline IV, moduleSlot=Moduleslot 1, channel=Reset pulscounter on channel 1}
      mask prompts: tsamp "Sample time"; contrType "Controller Type"; moduleSlot "Module slot"
      mask help: This block resets the pulsecounter from a specified input channel of the input module that is configured as a pulsecounter. A trigger on input pin 1 wil set the pulsecounter to the value applied on pin 2
      mask init:
      | % array with module slot infos
      | moduleSlotInfoStrings = {'Module Slot 1',  ...\
      | 						 'Module Slot 2',  ...\
      | 						 'Module Slot 3',  ...\
      | 						 'Module Slot 4',  ...\
      | 						 'Module Slot 5',  ...\
      | 						 'Module Slot 6',  ...\
      | 						 'Module Slot 7',  ...\
      | 						 'Module Slot 8'};
      | 
      | channelIDInfoStrings = {	'Input Channel 1',  ...\
      | 							'Input Channel 2',  ...\
      | 							'Input Channel 3',  ...\
      | 							'Input Channel 4',  ...\
      | 							'Input Channel 5',  ...\
      | 							'Input Channel 6',  ...\
      | 							'Input Channel 7',  ...\
      | 							'Input Channel 8',  ...\
      | 							'Input Channel 9',  ...\
      | 							'Input Channel 10'};
      | 
      | % construct the pinID info string
      | moduleSlotInfoStr = moduleSlotInfoStrings{moduleSlot};
      | inputChannelInfoStr  = channelIDInfoStrings{channel};
      | 
      | % Create resource keywords to be reserved in resource database
      | modelRTWFields = struct('moduleSlot', int2str(moduleSlot),'contrType', int2str(contrType),	'channel', int2str(channel));
      | 
      | set_param(gcb, 'RTWdata', modelRTWFields);
      mask TypeOptions contrType: GOcontroll Moduline IV | GOcontroll Moduline Mini | GOcontroll Moduline Display
      mask Callback contrType:
      | msk = Simulink.Mask.get(gcb);
      | p = msk.getParameter('moduleSlot');
      | 
      | func = get_param(gcb,'ContrType');
      | 
      | if(func == "GOcontroll Moduline IV")
      |     p.TypeOptions = {'Moduleslot 1','Moduleslot 2','Moduleslot 3','Moduleslot 4',...
      |                     'Moduleslot 5','Moduleslot 6','Moduleslot 7','Moduleslot 8'};
      | elseif (func == "GOcontroll Moduline Mini")
      |     p.TypeOptions = {'Moduleslot 1','Moduleslot 2','Moduleslot 3','Moduleslot 4'};
      | elseif (func == "GOcontroll Moduline Display")
      |     p.TypeOptions = {'Moduleslot 1','Moduleslot 2'};
      | end
      mask TypeOptions moduleSlot: Moduleslot 1 | Moduleslot 2 | Moduleslot 3 | Moduleslot 4 | Moduleslot 5 | Moduleslot 6 | Moduleslot 7 | Moduleslot 8
      mask TypeOptions channel: Reset pulscounter on channel 1 | Reset pulscounter on channel 2 | Reset pulscounter on channel 3 | Reset pulscounter on channel 4 | Reset pulscounter on channel 5 | Reset pulscounter on channel 6
      mask Display:
      | fprintf('Reset Pulse Counter\n%s\n%s', moduleSlotInfoStr, inputChannelInfoStr);
      | text(2, 6, ert_linux_target_version());
